simulink model "ieee9bus_wind_farm"  (R2015b)
settings: Solver=FixedStepAuto  StartTime=0.0  StopTime=40  FixedStep=Ts  RelTol=1e-3
values from neighbouring files (symbols this model uses):
  Cbase = 1/(100*pi*Xbase)    (= 6.0172001169e-06)    [ieee_9.m]
  Lbase = Xbase/(100*pi)    (= 1.68385929791)    [ieee_9.m]
  loadconnection = 15    [ieee_9.m]
  startup = 2    [ieee_9.m]
  Ts = 1e-5    (= 1e-05)    [ieee_9.m]
  Xbase = (Vbase^2)/Sbase    (= 529)    [ieee_9.m]
libraries: powerlib x125, powerlib_meascontrol x23, simulink x10, sps_avr x4, powerlib_extras x1
(part 1 of 2)
settings Model: SimulationMode=accelerator  Creator=Eren  LastModifiedBy=Eren

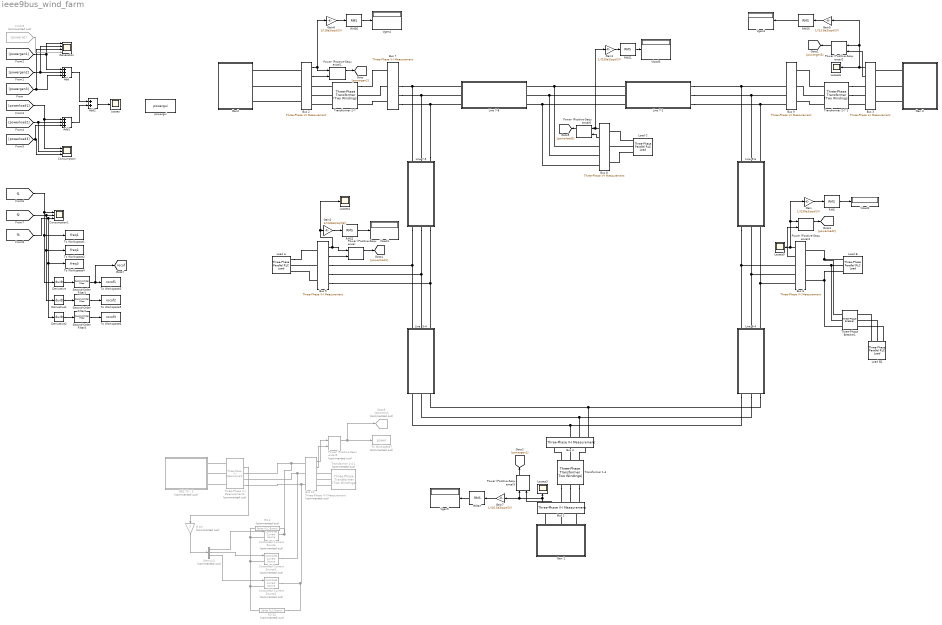
== system ieee9bus_wind_farm ==
  Add : Sum  Inputs=3
  Add1 : Sum  Inputs=3
  Add2 : Sum
  Bus {1..9} (9 alike) : powerlib/Measurements/Three-Phase V-I Measurement  VoltageMeasurement=phase-to-ground  SetLabelV=off  LabelV=Vsabc  Vpu=off  VpuLL=on  CurrentMeasurement=yes  SetLabelI=off  LabelI=Isabc  Ipu=off  Pbase=100e6  Vbase=690  OutputType=Complex  PhasorSimulation=off  PSBequivalent=0
  Bus 10 : powerlib/Measurements/Three-Phase V-I Measurement  Commented=on  VoltageMeasurement=phase-to-ground  SetLabelV=off  LabelV=Vsabc  Vpu=off  VpuLL=on  CurrentMeasurement=yes  SetLabelI=off  LabelI=Isabc  Ipu=off  Pbase=100e6  Vbase=690  OutputType=Complex  PhasorSimulation=off  PSBequivalent=0
  Concumption : Scope  NumInputPorts=3
  Concumption1 : Scope  NumInputPorts=3
  Controlled Current Source : powerlib/Electrical Sources/Controlled Current Source  Commented=on  Initialize=off  Source_Type=AC  Amplitude=0  Phase=0  Frequency=0  Measurements=None
  Controlled Current Source1 : powerlib/Electrical Sources/Controlled Current Source  Commented=on  Initialize=off  Source_Type=AC  Amplitude=0  Phase=0  Frequency=0  Measurements=None
  Controlled Current Source2 : powerlib/Electrical Sources/Controlled Current Source  Commented=on  Initialize=off  Source_Type=AC  Amplitude=0  Phase=0  Frequency=0  Measurements=None
  Demux3 : Demux  Commented=on  Outputs=3
  Derivative : Derivative
  Derivative1 : Derivative
  Derivative2 : Derivative
  From9 : From  Commented=on  GotoTag=powerwt
  G ain : Gain  Commented=on  Gain=7
  GE2.75 - 3 : Subsystem  Commented=on  mask{Prated=2.75e6, R=51.5, windspeed=9, Jtotal=1058.2, p=1.225, startuptime=5, winit=-160, gear=117.4, wmax=2*pi*(1735/60), fluxlinkage=4, pgen=2, Ld=10e-4, Lq=10.5e-4, Rs=1e-10, drivefreq=10e3, fnom=50, Srated=3.04e6, Vdcset=2500, Cdc=27e-3, Lfilter=2e-4, H=5, insup=25, supduration=2.5}
      mask prompts: Prated "Turbine Power (W)"; R "Blade Radius"; windspeed "Wind Speed"; Jtotal "Total Inertia"; p "Air Density"; startuptime "Turbine Start-up Time"; winit "Initial Generator Speed"; gear "Gearbox Ratio"; wmax "Max Generator Speed"; fluxlinkage "Flux Linkage"; pgen "Generator Pole Pairs"; Ld "Ld (H)"; Lq "Lq(H)"; Rs "Stator Resistance"; drivefreq "Drive Frequency"; fnom "Nominal Grid Frequency"; Srated "Drive Apparent Power"; Vdcset "DC Link Voltage"; Cdc "DC Link Capacitance"; Lfilter "Lfilter (H)"; H "Inertia Constant"; insup "Support Time"; supduration "Support Duration"
      mask Display: image(imread('gepic.jpg'))
  Gain : Gain  Gain=1/(230e3/sqrt(3))
  Gain1 : Gain  Gain=1/(230e3/sqrt(3))
  Gain2 : Gain  Gain=1/(230e3/sqrt(3))
  Gain5 : Gain  Gain=1/(13.8e3/sqrt(3))
  Gain6 : Gain  Gain=1/(18e3/sqrt(3))
  Gain7 : Gain  Gain=1/(16.5e3/sqrt(3))
  Gen 1 : Subsystem
  Gen 3 : Subsystem
  Gen2 : Subsystem
  "Generation " : Scope  NumInputPorts=4
  Goto6 : Goto  Commented=on  GotoTag=powerwt
  Line  5-4 : Subsystem
  Line 6-4 : Subsystem
  Line 7-1 : Subsystem
  Line 7-5 : Subsystem
  Line 7-8 : Subsystem
  Line 9-6 : Subsystem
  Load A : powerlib/Elements/Three-Phase Parallel RLC Load  LConnTagsString=A|B|C  Configuration=Y (grounded)  NominalVoltage=230e3  Vabc=[1e3 1e3 1e3]  Vabcp=[1e3 1e3 1e3]  NominalFrequency=50  UnbalancedPower=off  ActivePower=125e6  InductivePower=50e6  CapacitivePower=0  Pabc=[10e3 9e3 11e3]  QLabc=[100 90 110]  QCabc=[100 90 110]  Pabcp=[10e3 9e3 11e3]  QLabcp=[100 90 110]  QCabcp=[100 90 110]  Measurements=None  LoadType=constant PQ
  Load B : powerlib/Elements/Three-Phase Parallel RLC Load  LConnTagsString=A|B|C  Configuration=Y (grounded)  NominalVoltage=230e3  Vabc=[1e3 1e3 1e3]  Vabcp=[1e3 1e3 1e3]  NominalFrequency=50  UnbalancedPower=off  ActivePower=90e6  InductivePower=30e6  CapacitivePower=0  Pabc=[10e3 9e3 11e3]  QLabc=[100 90 110]  QCabc=[100 90 110]  Pabcp=[10e3 9e3 11e3]  QLabcp=[100 90 110]  QCabcp=[100 90 110]  Measurements=None  LoadType=constant PQ
  Load B2 : powerlib/Elements/Three-Phase Parallel RLC Load  LConnTagsString=A|B|C  Configuration=Y (grounded)  NominalVoltage=230e3  Vabc=[1e3 1e3 1e3]  Vabcp=[1e3 1e3 1e3]  NominalFrequency=50  UnbalancedPower=off  ActivePower=31.5e6  InductivePower=0  CapacitivePower=0  Pabc=[10e3 9e3 11e3]  QLabc=[100 90 110]  QCabc=[100 90 110]  Pabcp=[10e3 9e3 11e3]  QLabcp=[100 90 110]  QCabcp=[100 90 110]  Measurements=None  LoadType=constant PQ
  Load C : powerlib/Elements/Three-Phase Parallel RLC Load  LConnTagsString=A|B|C  Configuration=Y (grounded)  NominalVoltage=230e3  Vabc=[1e3 1e3 1e3]  Vabcp=[1e3 1e3 1e3]  NominalFrequency=50  UnbalancedPower=off  ActivePower=100e6  InductivePower=35e6  CapacitivePower=0  Pabc=[10e3 9e3 11e3]  QLabc=[100 90 110]  QCabc=[100 90 110]  Pabcp=[10e3 9e3 11e3]  QLabcp=[100 90 110]  QCabcp=[100 90 110]  Measurements=None  LoadType=constant PQ
  "Losses " : Scope
  Losses{3..6} (4 alike) : Scope
  Power (Positive-Sequence){,1..4,6} (6 alike) : powerlib_meascontrol/Measurements/Power (Positive-Sequence)  Freq=50  Vinit=[0, 0]  Iinit=[0, 0]  Ts=0
  Power (Positive-Sequence)5 : powerlib_meascontrol/Measurements/Power (Positive-Sequence)  Commented=on  Freq=50  Vinit=[0, 0]  Iinit=[0, 0]  Ts=0
  R2-2 : powerlib/Elements/Series RLC Branch  Commented=on  LConnTagsString=__new0  RConnTagsString=__new0  BranchType=R  Resistance=10000000000  Inductance=1e-3  SetiL0=off  InitialCurrent=0  Capacitance=1000000*Cbase  Setx0=off  InitialVoltage=0  Measurements=None
  R2-32 : powerlib/Elements/Series RLC Branch  Commented=on  LConnTagsString=__new0  RConnTagsString=__new0  BranchType=R  Resistance=10000000000  Inductance=1e-3  SetiL0=off  InitialCurrent=0  Capacitance=1000000*Cbase  Setx0=off  InitialVoltage=0  Measurements=None
  RMS{,1..2,5..7} (6 alike) : powerlib_meascontrol/Measurements/RMS  TrueRMS=on  Freq=50  RMSInit=120  Ts=0
  Second-Order Filter1 : powerlib_meascontrol/Filters/Second-Order Filter  FilterType=Lowpass  Fo=2  Zeta=0.707  Ts=0  Initialize=off  Vac_Init="[0,  0,  60]"  Vdc_Init=0  PlotResponse=off  FreqRange=[0, 500, 1]
  Second-Order Filter2 : powerlib_meascontrol/Filters/Second-Order Filter  FilterType=Lowpass  Fo=2  Zeta=0.707  Ts=0  Initialize=off  Vac_Init="[0,  0,  60]"  Vdc_Init=0  PlotResponse=off  FreqRange=[0, 500, 1]
  Second-Order Filter3 : powerlib_meascontrol/Filters/Second-Order Filter  FilterType=Lowpass  Fo=2  Zeta=0.707  Ts=0  Initialize=off  Vac_Init="[0,  0,  60]"  Vdc_Init=0  PlotResponse=off  FreqRange=[0, 500, 1]
  Three-Phase V-I Measurement1 : powerlib/Measurements/Three-Phase V-I Measurement  Commented=on  VoltageMeasurement=phase-to-ground  SetLabelV=off  LabelV=Vabc  Vpu=off  VpuLL=off  CurrentMeasurement=yes  SetLabelI=off  LabelI=Iabc  Ipu=off  Pbase=2.75e6  Vbase=690  OutputType=Complex  PhasorSimulation=off  PSBequivalent=0
  Three-Phase Breaker1 : powerlib/Elements/Three-Phase Breaker  InitialState=open  SwitchA=on  SwitchB=on  SwitchC=on  SwitchTimes=loadconnection  External=off  BreakerResistance=0.01  SnubberResistance=1e6  SnubberCapacitance=inf  Measurements=None
  To Workspace1 : ToWorkspace  VariableName=freq1  SaveFormat=Timeseries  SampleTime=-1
  To Workspace2 : ToWorkspace  VariableName=freq2  SaveFormat=Timeseries  SampleTime=-1
  To Workspace3 : ToWorkspace  VariableName=rocof1  SaveFormat=Timeseries  SampleTime=-1
  To Workspace4 : ToWorkspace  VariableName=freq3  SaveFormat=Timeseries  SampleTime=-1
  To Workspace5 : ToWorkspace  VariableName=rocof2  SaveFormat=Timeseries  SampleTime=-1
  To Workspace6 : ToWorkspace  VariableName=rocof3  SaveFormat=Timeseries  SampleTime=-1
  To Workspace7 : ToWorkspace  Commented=on  VariableName=power  SaveFormat=Structure With Time  SampleTime=-1
      settings: Decimation=3  Save2DSignal=2-D array (concatenate along first dimension)
  "Transformer 1-4 " : powerlib/Elements/Three-Phase Transformer (Two Windings)  Winding1Connection=Yg  Winding2Connection=Yg  CoreType=Three single-phase transformers  SetSaturation=off  Hysteresis=off  DataFile='hysteresis'  SetInitialFlux=off  Measurements=None  UNITS=pu  NominalPower=[ 250e6 , 50 ]  Winding1=[ 16.5e3 , 0.00001 , 0.0576/2 ]  Winding2="[ 230e3 , 0.00001  , 0.0576/2 ]"  Rm=500  Lm=500  L0=0.5  Saturation=[ 0,0 ; 0.0024,1.2 ; 1.0,1.52 ]  InitialFluxes=[ 0.8 , -0.8 , 0.7 ]  MoreParameters=off  BreakLoop=off  DataType=off  TransfoNumber=1
  Transformer 1-4 1 : powerlib/Elements/Three-Phase Transformer (Two Windings)  Commented=on  Winding1Connection=Yg  Winding2Connection=Yg  CoreType=Three single-phase transformers  SetSaturation=off  Hysteresis=off  DataFile='hysteresis'  SetInitialFlux=off  Measurements=None  UNITS=pu  NominalPower=[ 250e6 , 50 ]  Winding1=[ 690 , 0.00001 , 0.0576/2 ]  Winding2="[ 230e3 , 0.00001  , 0.0576/2 ]"  Rm=500  Lm=500  L0=0.5  Saturation=[ 0,0 ; 0.0024,1.2 ; 1.0,1.52 ]  InitialFluxes=[ 0.8 , -0.8 , 0.7 ]  MoreParameters=off  BreakLoop=off  DataType=off  TransfoNumber=1
  "Transformer 2-7 " : powerlib/Elements/Three-Phase Transformer (Two Windings)  Winding1Connection=Yg  Winding2Connection=Yg  CoreType=Three single-phase transformers  SetSaturation=off  Hysteresis=off  DataFile='hysteresis'  SetInitialFlux=off  Measurements=None  UNITS=pu  NominalPower=[ 250e6 , 50 ]  Winding1=[ 18e3 , 0 , 0 ]  Winding2="[ 230e3 , 0.00001  , 0.0625 ]"  Rm=500  Lm=500  L0=0.5  Saturation=[ 0,0 ; 0.0024,1.2 ; 1.0,1.52 ]  InitialFluxes=[ 0.8 , -0.8 , 0.7 ]  MoreParameters=off  BreakLoop=off  DataType=off  TransfoNumber=1
  Transformer 2-7 1 : powerlib/Elements/Three-Phase Transformer (Two Windings)  Winding1Connection=Yg  Winding2Connection=Yg  CoreType=Three single-phase transformers  SetSaturation=off  Hysteresis=off  DataFile='hysteresis'  SetInitialFlux=off  Measurements=None  UNITS=pu  NominalPower=[ 250e6 , 50 ]  Winding1=[ 13.8e3 , 0 , 0 ]  Winding2="[ 230e3 , 0.00001  , 0.0586 ]"  Rm=500  Lm=500  L0=0.5  Saturation=[ 0,0 ; 0.0024,1.2 ; 1.0,1.52 ]  InitialFluxes=[ 0.8 , -0.8 , 0.7 ]  MoreParameters=off  BreakLoop=off  DataType=off  TransfoNumber=1
  Vgen3 : Display
      settings: Decimation=5
  Vgen4 : Display
      settings: Decimation=5
  Vgen5 : Display
      settings: Decimation=5
  Vload1 : Display
      settings: Decimation=5
  Vload2 : Display
      settings: Decimation=5
  Vload3 : Display
      settings: Decimation=5
  powergui : powerlib/powergui  Priority=2  SimulationMode=Discrete  SolverType=Tustin  SampleTime=Ts  frequency=60  SPID=off  DisableSnubberDevices=off  DisableRonSwitches=off  DisableVfSwitches=off  SwTol=0  DisplayEquations=off  Interpol=off  ExternalGateDelay=off  methode=off  Ts=0  FunctionMessages=off  echomessages=off  HookPort=off  EnableUseOfTLC=off  x0status=blocks  frequencyindice=50  Pbase=100e6  ErrMax=1e-4  Iterations=50  UnitsV=kV  UnitsW=MW  buscounter=0  RestoreLinks=warning  ResistiveCurrentMeasurement=off  Frange=[0:2:500]  Ylog=off  Xlog=on  ShowGrid=off  save=off  variable=ZData  structure=0  ZoomFFT=on  StartTime=0.0  cycles=1  DisplayStyle=1  fundamental=60  FreqAxis=off  MaxFrequency=1000  frequencyindicesteady=1  RmsSteady=1  display=off
  tag scope: rocof=global
  wires:
  Bus 5/2 -> Power (Positive-Sequence)/2
  Power (Positive-Sequence)/1 -> [powerload1]
  Bus 6/1 -> Gain/1, Power (Positive-Sequence)4/1, Losses5/1
  Bus 2/2 -> Power (Positive-Sequence)1/2
  Bus 3/2 -> Power (Positive-Sequence)2/2
  Bus 1/2 -> Power (Positive-Sequence)3/2
  Power (Positive-Sequence)1/1 -> [powergen2]
  Power (Positive-Sequence)2/1 -> [powergen3]
  Power (Positive-Sequence)3/1 -> [powergen1]
  Bus 6/2 -> Power (Positive-Sequence)4/2
  Power (Positive-Sequence)4/1 -> [powerload2]
  [powergen1] -> "Generation "/1, Add/1
  [powergen2] -> Add/2, "Generation "/2
  [powergen3] -> "Generation "/3, Add/3
  [powerload1] -> Add1/1, Concumption/1
  [powerload2] -> Add1/2, Concumption/2
  [powerload3] -> Add1/3, Concumption/3
  Add/1 -> Add2/1
  Add1/1 -> Add2/2
  Add2/1 -> "Losses "/1
  Bus 8/2 -> Power (Positive-Sequence)6/2
  Power (Positive-Sequence)6/1 -> [powerload3]
  RMS/1 -> Vload2/1
  Gain/1 -> RMS/1
  Bus 8/1 -> Gain1/1, Power (Positive-Sequence)6/1
  RMS1/1 -> Vload3/1
  Gain1/1 -> RMS1/1
  Bus 5/1 -> Losses4/1, Gain2/1, Power (Positive-Sequence)/1
  RMS2/1 -> Vload1/1
  Gain2/1 -> RMS2/1
  Bus 1/1 -> Gain7/1, Power (Positive-Sequence)3/1, Losses3/1
  Bus 3/1 -> Gain5/1, Power (Positive-Sequence)2/1, Losses6/1
  [f2] -> Derivative1/1, To Workspace2/1, Concumption1/2
  [f1] -> Derivative/1, To Workspace1/1, Concumption1/1
  [f3] -> Derivative2/1, To Workspace4/1, Concumption1/3
  RMS6/1 -> Vgen4/1
  Gain6/1 -> RMS6/1
  Bus 2/1 -> Gain6/1, Power (Positive-Sequence)1/1
  RMS7/1 -> Vgen5/1
  Gain7/1 -> RMS7/1
  RMS5/1 -> Vgen3/1
  Gain5/1 -> RMS5/1
  Derivative/1 -> Second-Order Filter1/1
  Derivative1/1 -> Second-Order Filter2/1
  Derivative2/1 -> Second-Order Filter3/1
  Second-Order Filter1/1 -> [rocof], To Workspace3/1
  Second-Order Filter2/1 -> To Workspace5/1
  Second-Order Filter3/1 -> To Workspace6/1
  Bus 10/1 -> Power (Positive-Sequence)5/1
  Bus 10/2 -> Power (Positive-Sequence)5/2
  Demux3/1 -> Controlled Current Source/1
  Demux3/2 -> Controlled Current Source1/1
  Demux3/3 -> Controlled Current Source2/1
  Three-Phase V-I Measurement1/2 -> G ain/1
  G ain/1 -> Demux3/1
  Power (Positive-Sequence)5/1 -> Goto6/1, To Workspace7/1
  From9/1 -> "Generation "/4
  connections:
  Bus 5/RConn1 -- Line 7-5/RConn1 -- Line  5-4/LConn1
  Bus 5/RConn2 -- Line 7-5/RConn2 -- Line  5-4/LConn2
  Bus 5/RConn3 -- Line 7-5/RConn3 -- Line  5-4/LConn3
  Line 6-4/RConn1 -- Bus 4/RConn1 -- Line  5-4/RConn1
  Line  5-4/RConn2 -- Bus 4/RConn2 -- Line 6-4/RConn2
  Line 6-4/RConn3 -- Bus 4/RConn3 -- Line  5-4/RConn3
  Bus 6/RConn1 -- Line 9-6/RConn1 -- Line 6-4/LConn1
  Line 9-6/RConn3 -- Line 6-4/LConn3 -- Bus 6/RConn3
  Line 9-6/RConn2 -- Line 6-4/LConn2 -- Bus 6/RConn2
  Bus 9/RConn1 -- Line 7-1/RConn1 -- Line 9-6/LConn1
  Bus 9/RConn2 -- Line 7-1/RConn2 -- Line 9-6/LConn2
  Bus 9/RConn3 -- Line 7-1/RConn3 -- Line 9-6/LConn3
  Line 7-1/LConn1 -- Line 7-8/RConn1 -- Bus 8/RConn1
  Line 7-1/LConn2 -- Bus 8/RConn2 -- Line 7-8/RConn2
  Line 7-1/LConn3 -- Bus 8/RConn3 -- Line 7-8/RConn3
  Bus 7/RConn1 -- Line 7-8/LConn1 -- Line 7-5/LConn1
  Line 7-5/LConn2 -- Line 7-8/LConn2 -- Bus 7/RConn2
  Line 7-5/LConn3 -- Line 7-8/LConn3 -- Bus 7/RConn3
  Bus 2/LConn2 -- Gen2/RConn2
  Gen 3/RConn1 -- Bus 3/LConn1
  Bus 2/LConn1 -- Gen2/RConn1
  "Transformer 2-7 "/RConn1 -- Bus 7/LConn1
  "Transformer 1-4 "/LConn2 -- Bus 1/RConn2
  "Transformer 1-4 "/RConn1 -- Bus 4/LConn1
  "Transformer 1-4 "/RConn2 -- Bus 4/LConn2
  Bus 7/LConn3 -- "Transformer 2-7 "/RConn3
  Gen 1/RConn3 -- Bus 1/LConn3
  Bus 2/LConn3 -- Gen2/RConn3
  Gen 3/RConn3 -- Bus 3/LConn3
  "Transformer 2-7 "/LConn1 -- Bus 2/RConn1
  "Transformer 1-4 "/LConn3 -- Bus 1/RConn3
  Transformer 2-7 1/RConn2 -- Bus 9/LConn2
  Load A/LConn1 -- Bus 5/LConn1
  Load B/LConn2 -- Three-Phase Breaker1/LConn2 -- Bus 6/LConn2
  Bus 5/LConn2 -- Load A/LConn2
  Transformer 2-7 1/RConn3 -- Bus 9/LConn3
  Transformer 2-7 1/RConn1 -- Bus 9/LConn1
  Load B/LConn3 -- Three-Phase Breaker1/LConn3 -- Bus 6/LConn3
  "Transformer 2-7 "/LConn2 -- Bus 2/RConn2
  Load B/LConn1 -- Bus 6/LConn1 -- Three-Phase Breaker1/LConn1
  Gen 1/RConn2 -- Bus 1/LConn2
  Bus 5/LConn3 -- Load A/LConn3
  Transformer 2-7 1/LConn2 -- Bus 3/RConn2
  "Transformer 2-7 "/LConn3 -- Bus 2/RConn3
  Transformer 2-7 1/LConn1 -- Bus 3/RConn1
  Bus 7/LConn2 -- "Transformer 2-7 "/RConn2
  Gen 1/RConn1 -- Bus 1/LConn1
  Bus 4/LConn3 -- "Transformer 1-4 "/RConn3
  Gen 3/RConn2 -- Bus 3/LConn2
  "Transformer 1-4 "/LConn1 -- Bus 1/RConn1
  Bus 3/RConn3 -- Transformer 2-7 1/LConn3
  Load C/LConn1 -- Bus 8/LConn1
  Load C/LConn2 -- Bus 8/LConn2
  Load C/LConn3 -- Bus 8/LConn3
  Load B2/LConn1 -- Three-Phase Breaker1/RConn1
  Load B2/LConn3 -- Three-Phase Breaker1/RConn3
  Load B2/LConn2 -- Three-Phase Breaker1/RConn2
  Controlled Current Source/LConn1 -- R2-2/LConn1 -- Controlled Current Source1/LConn1 -- Controlled Current Source2/LConn1 -- R2-32/RConn1
  Controlled Current Source/RConn1 -- R2-2/RConn1 -- Three-Phase V-I Measurement1/RConn1 -- Bus 10/LConn1
  Controlled Current Source1/RConn1 -- Three-Phase V-I Measurement1/RConn2 -- Bus 10/LConn2
  Controlled Current Source2/RConn1 -- R2-32/LConn1 -- Bus 10/LConn3 -- Three-Phase V-I Measurement1/RConn3
  Three-Phase V-I Measurement1/LConn3 -- GE2.75 - 3/RConn3
  Three-Phase V-I Measurement1/LConn1 -- GE2.75 - 3/RConn1
  Three-Phase V-I Measurement1/LConn2 -- GE2.75 - 3/RConn2
  Transformer 1-4 1/LConn1 -- Bus 10/RConn1
  Transformer 1-4 1/LConn2 -- Bus 10/RConn2
  Transformer 1-4 1/LConn3 -- Bus 10/RConn3

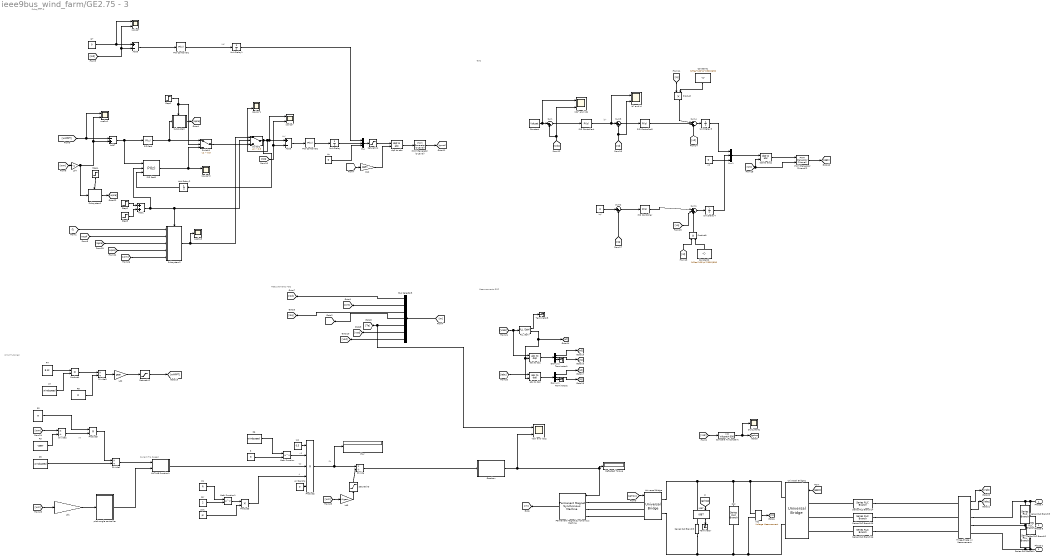
== system ieee9bus_wind_farm/GE2.75 - 3 ==
  note: Vd*
  note: Vq*
  note: Pt
  note: v3
  note: Cp
  note: A
  note: wt
  note: Current Tip Speed
  note: id*
  note: Measurements MSC
  note: GSC
  note: Measurements GSC
  note: Wind Turbine2
  note: Subsystem3
  1/2 : Constant  Value=0.5
  3 : Constant  Value=3
  Add1 : Sum
  Add3 : Sum  Inputs=+-
  Add5 : Sum  Inputs=+-
  Add7 : Sum  Inputs=-+
  Air Density : Constant  Value=p
  Bus Selector5 : BusSelector  OutputSignals=Stator current is_d (A),Rotor speed wm (rad/s),Stator current is_q (A),Rotor angle thetam (rad),Electromagnetic torque Te (N*m),Stator voltage Vs_q (V),Stator voltage Vs_d (V)
  Cdc : powerlib/Elements/Series RLC Branch  LConnTagsString=__new0  RConnTagsString=__new0  BranchType=C  Resistance=1  Inductance=1e-4  SetiL0=off  InitialCurrent=0  Capacitance=Cdc  Setx0=off  InitialVoltage=0  Measurements=None
  Compare To Constant : simulink/Logic and Bit Operations/Compare To Constant  relop=>=  const=Vdcset+300  OutDataTypeStr=boolean
  Constant : Constant  Value=Vdcset
  Constant1 : Constant  Value=(Lfilter*100*pi*2300)/690
  Constant2 : Constant  Value=(Lfilter*100*pi*2300)/690
  Dc Current1 : Scope
  Demux1 : Demux  Outputs=3
  Demux2 : Demux  Outputs=3
  Divide{,1..3} (4 alike) : Product  Inputs=*/
  Gearbox : Subsystem
  IGBT : powerlib/Power Electronics/IGBT  Ron=0.001  Lon=0  Vf=1  Tf=1e-6  Tt=2e-6  IC=0  Rs=1e5  Cs=inf  Measurements=on
  Id* : Constant  Value=0
  Ld1 : Gain  Gain=-pgen/(2*fnom*pi)
  Ld2 : Gain  Gain=gear
  Ld3 : Gain  Gain=-1/gear
  Ld4 : Gain  Gain=-1
  MATLAB Function1 : MATLAB Function  TreatAsAtomicUnit=on
  Math Function : Math  Operator=pow  SaturateOnIntegerOverflow=on
  Math Function1 : Math  Operator=pow  SaturateOnIntegerOverflow=on
  Mux : Mux  Inputs=3
  Mux1 : Mux  Inputs=3
  PID Controller : simulink/Continuous/PID Controller  Controller=PI  TimeDomain=Continuous-time  SampleTime=-1  IntegratorMethod=Forward Euler  FilterMethod=Forward Euler  Form=Parallel  UseFilter=on  ControllerParametersSource=internal  P=15  I=1  D=0  N=100  InitialConditionSource=internal  InitialConditionForIntegrator=0  InitialConditionForFilter=0  ExternalReset=none  LimitOutput=on  UpperSaturationLimit=2  LowerSaturationLimit=-2  LinearizeAsGain=on  AntiWindupMode=none  Kb=1  TrackingMode=off  Kt=1  PParamMin=[]  PParamMax=[]  IParamMin=[]  IParamMax=[]  DParamMin=[]  DParamMax=[]  NParamMin=[]  NParamMax=[]  KbParamMin=[]  KbParamMax=[]  KtParamMin=[]  KtParamMax=[]  POutMin=[]  POutMax=[]  IOutMin=[]  IOutMax=[]  DOutMin=[]  DOutMax=[]  NOutMin=[]  NOutMax=[]  KbOutMin=[]  KbOutMax=[]  KtOutMin=[]  KtOutMax=[]  IntegratorOutMin=[]  IntegratorOutMax=[]  FilterOutMin=[]  FilterOutMax=[]  SumOutMin=[]  SumOutMax=[]  SumI1OutMin=[]  SumI1OutMax=[]  SumI2OutMin=[]  SumI2OutMax=[]  SumI3OutMin=[]  SumI3OutMax=[]  SumDOutMin=[]  SumDOutMax=[]  SaturationOutMin=[]  SaturationOutMax=[]  IntegratorContinuousStateAttributes=''  IntegratorStateMustResolveToSignalObject=off  IntegratorRTWStateStorageClass=Auto  FilterContinuousStateAttributes=''  FilterStateMustResolveToSignalObject=off  FilterRTWStateStorageClass=Auto  DifferentiatorICPrevScaledInput=0  DifferentiatorOutMin=[]  DifferentiatorOutMax=[]
  PID Controller1 : simulink/Continuous/PID Controller  Controller=PI  TimeDomain=Discrete-time  SampleTime=Ts  IntegratorMethod=Forward Euler  FilterMethod=Forward Euler  Form=Parallel  UseFilter=on  ControllerParametersSource=internal  P=0.25  I=0.05  D=0  N=100  InitialConditionSource=internal  InitialConditionForIntegrator=0  InitialConditionForFilter=0  ExternalReset=none  LimitOutput=off  UpperSaturationLimit=inf  LowerSaturationLimit=-inf  LinearizeAsGain=on  AntiWindupMode=none  Kb=1  TrackingMode=off  Kt=1  PParamMin=[]  PParamMax=[]  IParamMin=[]  IParamMax=[]  DParamMin=[]  DParamMax=[]  NParamMin=[]  NParamMax=[]  KbParamMin=[]  KbParamMax=[]  KtParamMin=[]  KtParamMax=[]  POutMin=[]  POutMax=[]  IOutMin=[]  IOutMax=[]  DOutMin=[]  DOutMax=[]  NOutMin=[]  NOutMax=[]  KbOutMin=[]  KbOutMax=[]  KtOutMin=[]  KtOutMax=[]  IntegratorOutMin=[]  IntegratorOutMax=[]  FilterOutMin=[]  FilterOutMax=[]  SumOutMin=[]  SumOutMax=[]  SumI1OutMin=[]  SumI1OutMax=[]  SumI2OutMin=[]  SumI2OutMax=[]  SumI3OutMin=[]  SumI3OutMax=[]  SumDOutMin=[]  SumDOutMax=[]  SaturationOutMin=[]  SaturationOutMax=[]  IntegratorContinuousStateAttributes=''  IntegratorStateMustResolveToSignalObject=off  IntegratorRTWStateStorageClass=Auto  FilterContinuousStateAttributes=''  FilterStateMustResolveToSignalObject=off  FilterRTWStateStorageClass=Auto  DifferentiatorICPrevScaledInput=0  DifferentiatorOutMin=[]  DifferentiatorOutMax=[]
  PID Controller2 : simulink/Continuous/PID Controller  Controller=PI  TimeDomain=Discrete-time  SampleTime=Ts  IntegratorMethod=Forward Euler  FilterMethod=Forward Euler  Form=Parallel  UseFilter=on  ControllerParametersSource=internal  P=1  I=0.05  D=0  N=100  InitialConditionSource=internal  InitialConditionForIntegrator=0  InitialConditionForFilter=0  ExternalReset=none  LimitOutput=off  UpperSaturationLimit=inf  LowerSaturationLimit=-inf  LinearizeAsGain=on  AntiWindupMode=none  Kb=1  TrackingMode=off  Kt=1  PParamMin=[]  PParamMax=[]  IParamMin=[]  IParamMax=[]  DParamMin=[]  DParamMax=[]  NParamMin=[]  NParamMax=[]  KbParamMin=[]  KbParamMax=[]  KtParamMin=[]  KtParamMax=[]  POutMin=[]  POutMax=[]  IOutMin=[]  IOutMax=[]  DOutMin=[]  DOutMax=[]  NOutMin=[]  NOutMax=[]  KbOutMin=[]  KbOutMax=[]  KtOutMin=[]  KtOutMax=[]  IntegratorOutMin=[]  IntegratorOutMax=[]  FilterOutMin=[]  FilterOutMax=[]  SumOutMin=[]  SumOutMax=[]  SumI1OutMin=[]  SumI1OutMax=[]  SumI2OutMin=[]  SumI2OutMax=[]  SumI3OutMin=[]  SumI3OutMax=[]  SumDOutMin=[]  SumDOutMax=[]  SaturationOutMin=[]  SaturationOutMax=[]  IntegratorContinuousStateAttributes=''  IntegratorStateMustResolveToSignalObject=off  IntegratorRTWStateStorageClass=Auto  FilterContinuousStateAttributes=''  FilterStateMustResolveToSignalObject=off  FilterRTWStateStorageClass=Auto  DifferentiatorICPrevScaledInput=0  DifferentiatorOutMin=[]  DifferentiatorOutMax=[]
  PID Controller3 : simulink/Continuous/PID Controller  Controller=PI  TimeDomain=Continuous-time  SampleTime=-1  IntegratorMethod=Forward Euler  FilterMethod=Forward Euler  Form=Parallel  UseFilter=on  ControllerParametersSource=internal  P=100  I=5  D=0  N=100  InitialConditionSource=internal  InitialConditionForIntegrator=0  InitialConditionForFilter=0  ExternalReset=none  LimitOutput=on  UpperSaturationLimit=1.5  LowerSaturationLimit=-1.5  LinearizeAsGain=on  AntiWindupMode=none  Kb=1  TrackingMode=off  Kt=1  PParamMin=[]  PParamMax=[]  IParamMin=[]  IParamMax=[]  DParamMin=[]  DParamMax=[]  NParamMin=[]  NParamMax=[]  KbParamMin=[]  KbParamMax=[]  KtParamMin=[]  KtParamMax=[]  POutMin=[]  POutMax=[]  IOutMin=[]  IOutMax=[]  DOutMin=[]  DOutMax=[]  NOutMin=[]  NOutMax=[]  KbOutMin=[]  KbOutMax=[]  KtOutMin=[]  KtOutMax=[]  IntegratorOutMin=[]  IntegratorOutMax=[]  FilterOutMin=[]  FilterOutMax=[]  SumOutMin=[]  SumOutMax=[]  SumI1OutMin=[]  SumI1OutMax=[]  SumI2OutMin=[]  SumI2OutMax=[]  SumI3OutMin=[]  SumI3OutMax=[]  SumDOutMin=[]  SumDOutMax=[]  SaturationOutMin=[]  SaturationOutMax=[]  IntegratorContinuousStateAttributes=''  IntegratorStateMustResolveToSignalObject=off  IntegratorRTWStateStorageClass=Auto  FilterContinuousStateAttributes=''  FilterStateMustResolveToSignalObject=off  FilterRTWStateStorageClass=Auto  DifferentiatorICPrevScaledInput=0  DifferentiatorOutMin=[]  DifferentiatorOutMax=[]
  PID Controller4 : simulink/Continuous/PID Controller  Controller=PI  TimeDomain=Continuous-time  SampleTime=-1  IntegratorMethod=Forward Euler  FilterMethod=Forward Euler  Form=Parallel  UseFilter=on  ControllerParametersSource=internal  P=0.004  I=0.04  D=0  N=100  InitialConditionSource=internal  InitialConditionForIntegrator=0  InitialConditionForFilter=0  ExternalReset=none  LimitOutput=on  UpperSaturationLimit=1.2  LowerSaturationLimit=1e-6  LinearizeAsGain=on  AntiWindupMode=none  Kb=1  TrackingMode=off  Kt=1  PParamMin=[]  PParamMax=[]  IParamMin=[]  IParamMax=[]  DParamMin=[]  DParamMax=[]  NParamMin=[]  NParamMax=[]  KbParamMin=[]  KbParamMax=[]  KtParamMin=[]  KtParamMax=[]  POutMin=[]  POutMax=[]  IOutMin=[]  IOutMax=[]  DOutMin=[]  DOutMax=[]  NOutMin=[]  NOutMax=[]  KbOutMin=[]  KbOutMax=[]  KtOutMin=[]  KtOutMax=[]  IntegratorOutMin=[]  IntegratorOutMax=[]  FilterOutMin=[]  FilterOutMax=[]  SumOutMin=[]  SumOutMax=[]  SumI1OutMin=[]  SumI1OutMax=[]  SumI2OutMin=[]  SumI2OutMax=[]  SumI3OutMin=[]  SumI3OutMax=[]  SumDOutMin=[]  SumDOutMax=[]  SaturationOutMin=[]  SaturationOutMax=[]  IntegratorContinuousStateAttributes=''  IntegratorStateMustResolveToSignalObject=off  IntegratorRTWStateStorageClass=Auto  FilterContinuousStateAttributes=''  FilterStateMustResolveToSignalObject=off  FilterRTWStateStorageClass=Auto  DifferentiatorICPrevScaledInput=0  DifferentiatorOutMin=[]  DifferentiatorOutMax=[]
  PID fast : simulink/Continuous/PID Controller  Controller=PI  TimeDomain=Discrete-time  SampleTime=Ts  IntegratorMethod=Forward Euler  FilterMethod=Forward Euler  Form=Parallel  UseFilter=on  ControllerParametersSource=internal  P=750  I=1000  D=0  N=100  InitialConditionSource=internal  InitialConditionForIntegrator=0  InitialConditionForFilter=0  ExternalReset=none  LimitOutput=on  UpperSaturationLimit=1255  LowerSaturationLimit=200  LinearizeAsGain=on  AntiWindupMode=none  Kb=1  TrackingMode=off  Kt=1  PParamMin=[]  PParamMax=[]  IParamMin=[]  IParamMax=[]  DParamMin=[]  DParamMax=[]  NParamMin=[]  NParamMax=[]  KbParamMin=[]  KbParamMax=[]  KtParamMin=[]  KtParamMax=[]  POutMin=[]  POutMax=[]  IOutMin=[]  IOutMax=[]  DOutMin=[]  DOutMax=[]  NOutMin=[]  NOutMax=[]  KbOutMin=[]  KbOutMax=[]  KtOutMin=[]  KtOutMax=[]  IntegratorOutMin=[]  IntegratorOutMax=[]  FilterOutMin=[]  FilterOutMax=[]  SumOutMin=[]  SumOutMax=[]  SumI1OutMin=[]  SumI1OutMax=[]  SumI2OutMin=[]  SumI2OutMax=[]  SumI3OutMin=[]  SumI3OutMax=[]  SumDOutMin=[]  SumDOutMax=[]  SaturationOutMin=[]  SaturationOutMax=[]  IntegratorContinuousStateAttributes=''  IntegratorStateMustResolveToSignalObject=off  IntegratorRTWStateStorageClass=Auto  FilterContinuousStateAttributes=''  FilterStateMustResolveToSignalObject=off  FilterRTWStateStorageClass=Auto  DifferentiatorICPrevScaledInput=0  DifferentiatorOutMin=[]  DifferentiatorOutMax=[]
  PID fast1 : simulink/Continuous/PID Controller  Controller=PI  TimeDomain=Discrete-time  SampleTime=Ts  IntegratorMethod=Forward Euler  FilterMethod=Forward Euler  Form=Parallel  UseFilter=on  ControllerParametersSource=internal  P=45  I=9  D=0  N=100  InitialConditionSource=external  InitialConditionForIntegrator=0  InitialConditionForFilter=0  ExternalReset=falling  LimitOutput=on  UpperSaturationLimit=1255  LowerSaturationLimit=200  LinearizeAsGain=on  AntiWindupMode=none  Kb=1  TrackingMode=off  Kt=1  PParamMin=[]  PParamMax=[]  IParamMin=[]  IParamMax=[]  DParamMin=[]  DParamMax=[]  NParamMin=[]  NParamMax=[]  KbParamMin=[]  KbParamMax=[]  KtParamMin=[]  KtParamMax=[]  POutMin=[]  POutMax=[]  IOutMin=[]  IOutMax=[]  DOutMin=[]  DOutMax=[]  NOutMin=[]  NOutMax=[]  KbOutMin=[]  KbOutMax=[]  KtOutMin=[]  KtOutMax=[]  IntegratorOutMin=[]  IntegratorOutMax=[]  FilterOutMin=[]  FilterOutMax=[]  SumOutMin=[]  SumOutMax=[]  SumI1OutMin=[]  SumI1OutMax=[]  SumI2OutMin=[]  SumI2OutMax=[]  SumI3OutMin=[]  SumI3OutMax=[]  SumDOutMin=[]  SumDOutMax=[]  SaturationOutMin=[]  SaturationOutMax=[]  IntegratorContinuousStateAttributes=''  IntegratorStateMustResolveToSignalObject=off  IntegratorRTWStateStorageClass=Auto  FilterContinuousStateAttributes=''  FilterStateMustResolveToSignalObject=off  FilterRTWStateStorageClass=Auto  DifferentiatorICPrevScaledInput=0  DifferentiatorOutMin=[]  DifferentiatorOutMax=[]
  PLL (3ph) : powerlib_meascontrol/PLL/PLL (3ph)  Fmin=45  Par_Init=[0, 50]  ParK=[180, 3200, 1]  TcD=1e-4  MaxRateChangeFreq=12  FilterCutOffFreq=25  Ts=Ts  AGC=on
  PWM Generator (2-Level) : powerlib_meascontrol/Pulse & Signal Generators/PWM Generator (2-Level)  ModulatorType=Three-phase bridge (6 pulses)  ModulatorMode=Unsynchronized  Fc=drivefreq  Pc=90  nF=60  MinMax="[ -1  1 ]"  SamplingTechnique=Natural  ModulatingSignals=off  m=0.8  Freq=60  Phase=0  Ts=Ts  ShowCarrierOutport=off
  PWM Generator (2-Level)2 : powerlib_meascontrol/Pulse & Signal Generators/PWM Generator (2-Level)  ModulatorType=Three-phase bridge (6 pulses)  ModulatorMode=Synchronized  Fc=50*60  Pc=90  nF=500  MinMax="[ -1  1 ]"  SamplingTechnique=Natural  ModulatingSignals=off  m=0.8  Freq=60  Phase=0  Ts=Ts  ShowCarrierOutport=off
  Permanent Magnet Synchronous Machine : powerlib/Machines/Permanent Magnet Synchronous Machine  NbPhases=3  FluxDistribution=Sinusoidal  RotorType=Round  MechanicalLoad=Torque Tm  PresetModel=No  ShowDetailedParameters=on  MeasurementBus=off  Resistance=Rs  Inductance=8.5e-3  dqInductances=[Ld,Lq]  La=Lq  MachineConstant=Flux linkage established by magnets (V.s)  Flux=fluxlinkage  VoltageCst=1451.0395  TorqueCst=12  Flat=120  Mechanical=[Jtotal 1.349e-05 pgen 0]  PolePairs=2  InitialConditions=[winit,0, 0,0]  InitialConditions5ph=[0 0 0 0 0 0]  TsPowergui=0  TsBlock=-1  RefAngle=Aligned with phase A axis (original Park)
  Pp2 : Gain  Gain=pgen
  Product{,1,3..5} (5 alike) : Product
  Product2 : Product  Inputs=5
  Ptur : Display
  R1 : Constant  Value=R
  R2 : Constant  Value=R
  R3 : Constant  Value=-gear
  R4 : Constant  Value=8.12
  R5 : Constant  Value=windspeed
  R6 : Constant  Value=windspeed
  R7 : Constant  Value=windspeed
  R8 : Constant  Value=R
  Reflected Torque : Display
  Saturatin1 : Saturate  UpperLimit=2000  LowerLimit=-2000
  Saturatin2 : Saturate  UpperLimit=wmax  LowerLimit=1e-8
  Saturatin3 : Saturate  UpperLimit=inf  LowerLimit=1e-8
  Series RLC Branch1 : powerlib/Elements/Series RLC Branch  LConnTagsString=__new0  RConnTagsString=__new0  BranchType=R  Resistance=1e10  Inductance=Lfilter  SetiL0=off  InitialCurrent=0  Capacitance=1e-6  Setx0=off  InitialVoltage=0  Measurements=None
  Series RLC Branch14 : powerlib/Elements/Series RLC Branch  LConnTagsString=__new0  RConnTagsString=__new0  BranchType=L  Resistance=1  Inductance=Lfilter  SetiL0=off  InitialCurrent=0  Capacitance=1e-6  Setx0=off  InitialVoltage=0  Measurements=None
  Series RLC Branch15 : powerlib/Elements/Series RLC Branch  LConnTagsString=__new0  RConnTagsString=__new0  BranchType=L  Resistance=1  Inductance=Lfilter  SetiL0=off  InitialCurrent=0  Capacitance=1e-6  Setx0=off  InitialVoltage=0  Measurements=None
  Series RLC Branch16 : powerlib/Elements/Series RLC Branch  LConnTagsString=__new0  RConnTagsString=__new0  BranchType=L  Resistance=1  Inductance=Lfilter  SetiL0=off  InitialCurrent=0  Capacitance=1e-6  Setx0=off  InitialVoltage=0  Measurements=None
  Series RLC Branch2 : powerlib/Elements/Series RLC Branch  LConnTagsString=__new0  RConnTagsString=__new0  BranchType=R  Resistance=1e10  Inductance=Lfilter  SetiL0=off  InitialCurrent=0  Capacitance=1e-6  Setx0=off  InitialVoltage=0  Measurements=None
  Series RLC Branch3 : powerlib/Elements/Series RLC Branch  LConnTagsString=__new0  RConnTagsString=__new0  BranchType=R  Resistance=1  Inductance=1e-4  SetiL0=off  InitialCurrent=0  Capacitance=Cdc  Setx0=off  InitialVoltage=0  Measurements=None
  Series RLC Branch5 : powerlib/Elements/Series RLC Branch  LConnTagsString=__new0  RConnTagsString=__new0  BranchType=R  Resistance=1e10  Inductance=Lfilter  SetiL0=off  InitialCurrent=0  Capacitance=1e-6  Setx0=off  InitialVoltage=0  Measurements=None
  Step1 : Step  Time=insup  Before=1  After=0  SampleTime=Ts
  Step2 : Step  Time=insup  SampleTime=Ts
  Step4 : Step  Time=insup  Before=1  After=0  SampleTime=Ts
  Step5 : Step  Time=insup+supduration  After=-1  SampleTime=Ts
  Subsystem : Subsystem
  Subsystem1 : Subsystem
  Subsystem2 : Subsystem
  Sum : Sum  Inputs=|-+
  Sum1 : Sum  Inputs=|+++
  Sum2 : Sum  Inputs=|+-
  Sum3 : Sum  Inputs=|+-
  Sum4 : Sum  Inputs=|-++
  Switch1 : Switch  Criteria=u2 > Threshold  Threshold=0.5
  Switch2 : Switch  Criteria=u2 > Threshold  Threshold=0.5
  Terminator{,1..3} (4 alike) : Terminator
  Three-Phase V-I Measurement : powerlib/Measurements/Three-Phase V-I Measurement  VoltageMeasurement=phase-to-ground  SetLabelV=off  LabelV=Vabc  Vpu=on  VpuLL=off  CurrentMeasurement=yes  SetLabelI=off  LabelI=Iabc  Ipu=on  Pbase=2.75e6  Vbase=690  OutputType=Complex  PhasorSimulation=off  PSBequivalent=0
  Unit Delay{,1..4} (5 alike) : UnitDelay  SampleTime=Ts
  Universal Bridge : powerlib/Power Electronics/Universal Bridge  Arms=3  SnubberResistance=1e5  SnubberCapacitance=inf  Device=IGBT / Diodes  Ron=1e-3  Lon=0  ForwardVoltages="[  0  0  ]"  ForwardVoltage=0  GTOparameters=[ 10e-6 , 20e-6 ]  IGBTparameters=[ 1e-6 , 2e-6 ]  Measurements=None  Measurements_2=None  converterType=Rectifier
  Universal Bridge1 : powerlib/Power Electronics/Universal Bridge  Arms=3  SnubberResistance=1e5  SnubberCapacitance=inf  Device=IGBT / Diodes  Ron=0.00001  Lon=0  ForwardVoltages="[  0  0  ]"  ForwardVoltage=0  GTOparameters=[ 10e-6 , 20e-6 ]  IGBTparameters=[ 0 , 0 ]  Measurements=None  Measurements_2=None  converterType=Rectifier
  Vdc : powerlib/Measurements/Voltage Measurement  PhasorSimulation=off  OutputType=Complex  PSBequivalent=0
  Vdc* and Vdc : Scope  NumInputPorts=2
  Vdc* and Vdc2 : Scope  NumInputPorts=2
  Vo : Constant  Value=0
  abc to dq1 : powerlib_meascontrol/Transformations/abc to dq0  Alignment=90 degrees behind phase A axis
  abc to dq2 : powerlib_meascontrol/Transformations/abc to dq0  Alignment=90 degrees behind phase A axis
  dq0 to abc : powerlib_meascontrol/Transformations/dq0 to abc  Alignment=Aligned with phase A axis
  dq0 to abc1 : powerlib_meascontrol/Transformations/dq0 to abc  Alignment=90 degrees behind phase A axis
  "id* and id " : Scope  NumInputPorts=2
  iq* : Constant  Value=0
  isd-isd* : Scope  NumInputPorts=2
  isq-isq* : Scope  NumInputPorts=2
  isq-isq*1 : Scope  NumInputPorts=2
  isq-isq*2 : Scope  NumInputPorts=2
  pitch angle controller : Subsystem
  sqr : Constant  Value=2
  sqr1 : Constant  Value=pi
  v0 : Constant  Value=0
  wref-w1 : Scope  NumInputPorts=2
  wref-w3 : Scope
  Phase A : PMIOPort  Port=1  Side=Right
  Phase B : PMIOPort  Port=2  Side=Right
  Phase C : PMIOPort  Port=3  Side=Right
  wires:
  Ld4/1 -> wref-w1/2, Add7/2, Subsystem1/1(In1)
  [wm] -> Ld4/1
  PID fast/1 -> Switch1/1, Subsystem/1(In1)
  PWM Generator (2-Level)/1 -> [gmsc]
  dq0 to abc/1 -> PWM Generator (2-Level)/1
  Vo/1 -> Mux/3
  Mux/1 -> Saturatin1/1
  Add3/1 -> PID Controller2/1
  Add7/1 -> PID fast1/1, PID fast/1
  Add5/1 -> PID Controller1/1
  [wMPPT] -> Add7/1, wref-w1/1
  PID Controller2/1 -> Unit Delay/1
  Id*/1 -> isd-isd*/1, Add5/1
  Saturatin1/1 -> dq0 to abc/1
  [isd] -> Add5/2, isd-isd*/2
  Pp2/1 -> dq0 to abc/2
  [isq] -> Add3/2, isq-isq*/2
  Unit Delay1/1 -> Mux/1
  [thetam] -> Pp2/1
  PID Controller1/1 -> Unit Delay1/1
  Unit Delay/1 -> Mux/2
  Subsystem1/1(Out1) -> [wpre]
  Step4/1 -> Subsystem1/Enable
  [f1] -> Subsystem2/1(In1)
  Subsystem/1(Out1) -> [iqpre]
  Switch2/1 -> Unit Delay2/1, isq-isq*1/2, Add3/1, isq-isq*/1
  [wm] -> Subsystem2/5(In5)
  [iqpre] -> Subsystem2/3(In3)
  [rocof] -> Subsystem2/2(In2)
  [wpre] -> Subsystem2/4(In4)
  Demux1/3 -> Terminator2/1
  Demux2/3 -> Terminator1/1
  Three-Phase V-I Measurement/2 -> [Iabc]
  Three-Phase V-I Measurement/1 -> [Vabc]
  Air Density/1 -> Product2/5
  1/2/1 -> Product2/1
  Product3/1 -> Product2/4
  Math Function1/1 -> Product3/1
  sqr1/1 -> Product3/2
  [wm] -> Ld3/1
  Math Function/1 -> Product2/2
  sqr/1 -> Math Function1/2
  R1/1 -> Math Function1/1
  3/1 -> Math Function/2
  R2/1 -> Product5/1
  [wm] -> Divide2/1
  Product5/1 -> Divide1/1
  R5/1 -> Divide1/2
  Divide1/1 -> MATLAB Function1/1(u)
  Divide2/1 -> Product5/2
  Ld3/1 -> Saturatin3/1
  MATLAB Function1/1(Cp) -> Product2/3
  R3/1 -> Divide2/2
  R6/1 -> Math Function/1
  pitch angle controller/1(Beta) -> MATLAB Function1/2(B)
  Product2/1 -> Divide/1, Ptur/1
  Ld1/1 -> pitch angle controller/1(wr)
  [wm] -> Ld1/1
  Saturatin3/1 -> Divide/2
  R4/1 -> Product4/1
  R7/1 -> Product4/2
  Product4/1 -> Divide3/1
  R8/1 -> Divide3/2
  Divide3/1 -> Ld2/1
  Ld2/1 -> Saturatin2/1
  Saturatin2/1 -> [wMPPT]
  [Vabc] -> PLL (3ph)/1, abc to dq1/1
  PLL (3ph)/2 -> [wt], abc to dq1/2, abc to dq2/2
  [Iabc] -> abc to dq2/1
  Demux2/1 -> [vd]
  Demux2/2 -> [vq]
  Demux1/1 -> [id]
  Demux1/2 -> [iq]
  abc to dq1/1 -> Demux2/1
  abc to dq2/1 -> Demux1/1
  PWM Generator (2-Level)2/1 -> [ggsc]
  iq*/1 -> Sum2/1
  Sum3/1 -> PID Controller3/1
  PID Controller4/1 -> Sum3/1, "id* and id "/1
  PID Controller/1 -> Sum1/1
  [vq] -> Sum1/2
  Sum2/1 -> PID Controller/1
  PID Controller3/1 -> Sum4/2
  Sum4/1 -> Unit Delay3/1
  Mux1/1 -> dq0 to abc1/1
  [wt] -> PWM Generator (2-Level)2/2, dq0 to abc1/2
  Sum1/1 -> Unit Delay4/1
  v0/1 -> Mux1/3
  [Vdc] -> Sum/2, Vdc* and Vdc/2
  Sum/1 -> PID Controller4/1
  dq0 to abc1/1 -> PWM Generator (2-Level)2/1
  Constant/1 -> Sum/1, Vdc* and Vdc/1
  Unit Delay3/1 -> Mux1/1
  Unit Delay4/1 -> Mux1/2
  [vd] -> Sum4/3
  [iq] -> Product/1
  Constant1/1 -> Product/2
  [id] -> Product1/1
  Constant2/1 -> Product1/2
  [iq] -> Sum2/2
  [id] -> Sum3/2, "id* and id "/2
  Product/1 -> Sum4/1
  Product1/1 -> Sum1/3
  Bus Selector5/6 -> [vsq]  "<Stator voltage Vs_q (V)>"
  Bus Selector5/2 -> [wm]  "<Rotor speed wm (rad/s)>"
  Bus Selector5/5 -> Vdc* and Vdc2/1, [Te]  "<Electromagnetic torque Te (N*m)>"
  Bus Selector5/4 -> [thetam]  "<Rotor angle thetam (rad)>"
  Bus Selector5/1 -> [isd]  "<Stator current is_d (A)>"
  Bus Selector5/3 -> [isq]  "<Stator current is_q (A)>"
  Bus Selector5/7 -> [vsd]  "<Stator voltage Vs_d (V)>"
  [m] -> Bus Selector5/1
  Permanent Magnet Synchronous Machine/1 -> [m]
  [gmsc] -> Universal Bridge/1
  IGBT/1 -> Terminator/1
  [gchop] -> IGBT/1
  Compare To Constant/1 -> [gchop], Dc Current1/1
  [Vdc] -> Compare To Constant/1
  Vdc/1 -> [Vdc]
  [ggsc] -> Universal Bridge1/1
  Divide/1 -> Gearbox/1(Tt)
  Gearbox/1(Tt') -> Vdc* and Vdc2/2, Reflected Torque/1, Permanent Magnet Synchronous Machine/1
  PLL (3ph)/1 -> Terminator3/1
  Step1/1 -> Switch1/2, Subsystem/Enable
  Step5/1 -> Add1/2
  Step2/1 -> Add1/1
  Add1/1 -> PID fast1/2, Subsystem2/Enable, Switch2/2
  Subsystem2/1(Out1) -> Switch2/1, wref-w3/1
  Switch1/1 -> Switch2/3
  PID fast1/1 -> Switch1/3, isq-isq*2/1
  Unit Delay2/1 -> PID fast1/3
  connections:
  Series RLC Branch3/LConn1 -- IGBT/RConn1
  Cdc/LConn1 -- Vdc/LConn1 -- Universal Bridge1/RConn1 -- IGBT/LConn1 -- Universal Bridge/RConn1
  Series RLC Branch14/LConn1 -- Universal Bridge1/LConn1
  Series RLC Branch15/LConn1 -- Universal Bridge1/LConn2
  Permanent Magnet Synchronous Machine/LConn3 -- Universal Bridge/LConn3
  Vdc/LConn2 -- Cdc/RConn1 -- Series RLC Branch3/RConn1 -- Universal Bridge/RConn2 -- Universal Bridge1/RConn2
  Series RLC Branch15/RConn1 -- Three-Phase V-I Measurement/LConn2
  Series RLC Branch16/LConn1 -- Universal Bridge1/LConn3
  Series RLC Branch16/RConn1 -- Three-Phase V-I Measurement/LConn3
  Series RLC Branch14/RConn1 -- Three-Phase V-I Measurement/LConn1
  Permanent Magnet Synchronous Machine/LConn2 -- Universal Bridge/LConn2
  Permanent Magnet Synchronous Machine/LConn1 -- Universal Bridge/LConn1
  Phase C/RConn1 -- Series RLC Branch2/RConn1 -- Series RLC Branch1/RConn1 -- Three-Phase V-I Measurement/RConn3
  Three-Phase V-I Measurement/RConn1 -- Series RLC Branch5/LConn1 -- Series RLC Branch2/LConn1 -- Phase A/RConn1
  Three-Phase V-I Measurement/RConn2 -- Series RLC Branch1/LConn1 -- Series RLC Branch5/RConn1 -- Phase B/RConn1
